simulink model "Overcurrent_Relay_design"  (R2024b)
settings: Solver=VariableStepAuto  StartTime=0.0  StopTime=0.4  RelTol=1e-3
undefined symbols (not defined in the file): D1, Delta
libraries: spsFourierLib x9, simulink x6, spsThreePhasePISectionLineLib x3, spsThreePhaseParallelRLCLoadLib x3, spsThreePhaseVIMeasurementLib x3, spsOnDelayLib x2, simulink_extras x2, spsThreePhaseBreakerLib x2, spsThreePhaseFaultLib x2, spsThreePhaseTransformerTwoWindingsLib x1, spsThreePhaseSourceLib x1, sps_lib x1
settings Model: Creator=Sabyasachi  LastModifiedBy=Sabyasachi

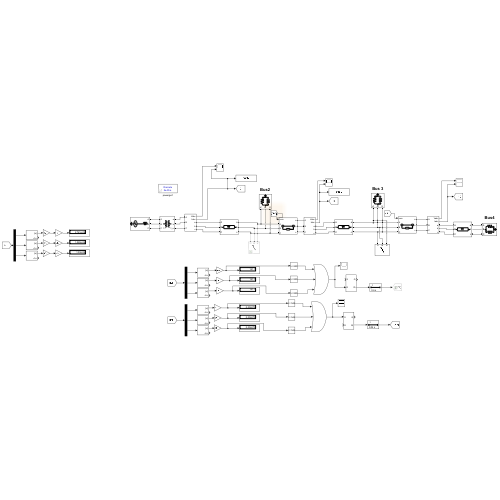
[thumbnail: Simulink's stored preview of the top-level diagram]
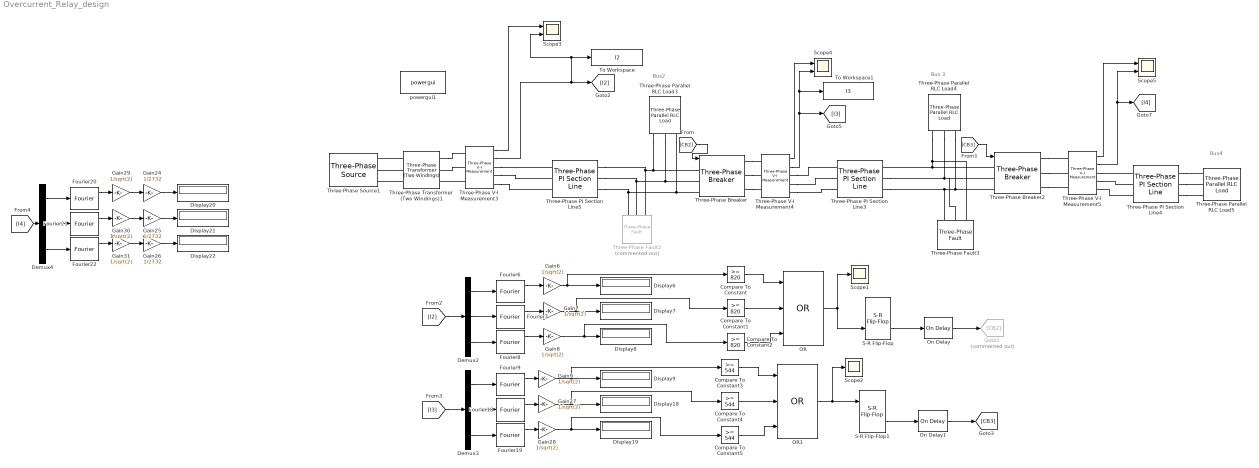
== system Overcurrent_Relay_design ==
  note: Bus4
  note: Bus 3
  note: Bus2
  Compare To Constant : simulink/Logic and Bit Operations/Compare To Constant  relop=>=  const=820  OutDataTypeStr=boolean
  Compare To Constant1 : simulink/Logic and Bit Operations/Compare To Constant  relop=>=  const=820  OutDataTypeStr=boolean
  Compare To Constant2 : simulink/Logic and Bit Operations/Compare To Constant  relop=>=  const=820  OutDataTypeStr=boolean
  Compare To Constant3 : simulink/Logic and Bit Operations/Compare To Constant  relop=>=  const=544  OutDataTypeStr=boolean
  Compare To Constant4 : simulink/Logic and Bit Operations/Compare To Constant  relop=>=  const=544  OutDataTypeStr=boolean
  Compare To Constant5 : simulink/Logic and Bit Operations/Compare To Constant  relop=>=  const=544  OutDataTypeStr=boolean
  Demux2 : Demux  Outputs=3
  Demux3 : Demux  Outputs=3
  Demux4 : Demux  Outputs=3
  Display{6..9,18..22} (9 alike) : Display
  Fourier{6..9,18..22} (9 alike) : spsFourierLib/Fourier  Freq=50  n=1  InInit=[0, 0]  Ts=0
  Gain24 : Gain  Gain=1/2732
  Gain25 : Gain  Gain=1/2732
  Gain26 : Gain  Gain=1/2732
  Gain{6..9,27..31} (9 alike) : Gain  Gain=1/sqrt(2)
  Goto1 : Goto  Commented=on  GotoTag=CB2
  OR : Logic  Operator=OR  Inputs=3  IconShape=distinctive  AllPortsSameDT=off  OutDataTypeStr=boolean
  OR1 : Logic  Operator=OR  Inputs=3  IconShape=distinctive  AllPortsSameDT=off  OutDataTypeStr=boolean
  On Delay : spsOnDelayLib/On Delay  DelayType=On delay  delay=0.6  ic=0  Ts=0
  On Delay1 : spsOnDelayLib/On Delay  DelayType=On delay  delay=0.04  ic=0  Ts=0
  S-R Flip-Flop : simulink_extras/Flip Flops/S-R Flip-Flop  initial_condition=0
  S-R Flip-Flop1 : simulink_extras/Flip Flops/S-R Flip-Flop  initial_condition=0
  Scope1 : Scope
  Scope2 : Scope
  Scope3 : Scope  NumInputPorts=2
  Scope4 : Scope  NumInputPorts=2
  Scope5 : Scope  NumInputPorts=2
  Three-Phase PI Section Line3 : spsThreePhasePISectionLineLib/Three-Phase PI Section Line  LConnTagsString=a|b|c  RConnTagsString=A|B|C  Length=1  Frequency=50  Resistances=[0.1486 0.2972]  Inductances=[4.73e-4 9.46e-4]  Capacitances=[1e-12 1e-12]
  Three-Phase PI Section Line4 : spsThreePhasePISectionLineLib/Three-Phase PI Section Line  LConnTagsString=a|b|c  RConnTagsString=A|B|C  Length=1  Frequency=50  Resistances=[0.1486 0.2972]  Inductances=[4.73e-4 9.46e-4]  Capacitances=[1e-12 1e-12]
  Three-Phase PI Section Line5 : spsThreePhasePISectionLineLib/Three-Phase PI Section Line  LConnTagsString=a|b|c  RConnTagsString=A|B|C  Length=1  Frequency=50  Resistances=[0.1486 0.2972]  Inductances=[4.73e-4 9.46e-4]  Capacitances=[1e-12 1e-12]
  Three-Phase Parallel RLC Load3 : spsThreePhaseParallelRLCLoadLib/Three-Phase Parallel RLC Load  LConnTagsString=A|B|C  Configuration=Y (grounded)  NominalVoltage=11e3  Vabc=[1e3 1e3 1e3]  Vabcp=[1e3 1e3 1e3]  NominalFrequency=50  UnbalancedPower=off  ActivePower=2.42e6  InductivePower=1.245e6  CapacitivePower=0  Pabc=[10e3 9e3 11e3]  QLabc=[100 90 110]  QCabc=[100 90 110]  Pabcp=[10e3 9e3 11e3]  QLabcp=[100 90 110]  QCabcp=[100 90 110]  Measurements=None  LoadType=constant Z
  Three-Phase Parallel RLC Load4 : spsThreePhaseParallelRLCLoadLib/Three-Phase Parallel RLC Load  LConnTagsString=A|B|C  Configuration=Y (grounded)  NominalVoltage=11e3  Vabc=[1e3 1e3 1e3]  Vabcp=[1e3 1e3 1e3]  NominalFrequency=50  UnbalancedPower=off  ActivePower=1.61e6  InductivePower=0.830e6  CapacitivePower=0  Pabc=[10e3 9e3 11e3]  QLabc=[100 90 110]  QCabc=[100 90 110]  Pabcp=[10e3 9e3 11e3]  QLabcp=[100 90 110]  QCabcp=[100 90 110]  Measurements=None  LoadType=constant Z
  Three-Phase Parallel RLC Load5 : spsThreePhaseParallelRLCLoadLib/Three-Phase Parallel RLC Load  LConnTagsString=A|B|C  Configuration=Y (grounded)  NominalVoltage=11e3  Vabc=[1e3 1e3 1e3]  Vabcp=[1e3 1e3 1e3]  NominalFrequency=50  UnbalancedPower=off  ActivePower=3.23e6  InductivePower=1.660e6  CapacitivePower=0  Pabc=[10e3 9e3 11e3]  QLabc=[100 90 110]  QCabc=[100 90 110]  Pabcp=[10e3 9e3 11e3]  QLabcp=[100 90 110]  QCabcp=[100 90 110]  Measurements=None  LoadType=constant Z
  Three-Phase Transformer (Two Windings)1 : spsThreePhaseTransformerTwoWindingsLib/Three-Phase Transformer (Two Windings)  Winding1Connection=Delta (D1)  Winding2Connection=Yg  CoreType=Three single-phase transformers  SetSaturation=off  Hysteresis=off  DataFile='hysteresis'  SetInitialFlux=off  Measurements=None  UNITS=pu  NominalPower=[ 17e6 , 50 ]  Winding1=[33e3 , 1e-6 , 0.05 ]  Winding2=[ 11e3 , 1e-6 , 1e-6 ]  Rm=500  Lm=500  L0=0.5  Saturation=[ 0,0 ; 0.0024,1.2 ; 1.0,1.52 ]  InitialFluxes=[ 0.8 , -0.8 , 0.7 ]  BreakLoop=off  DiscreteSolver=Trapezoidal iterative  DataType=off  TransfoNumber=1
  Three-Phase V-I Measurement3 : spsThreePhaseVIMeasurementLib/Three-Phase V-I Measurement  VoltageMeasurement=phase-to-ground  SetLabelV=off  LabelV=Vabc  Vpu=off  VpuLL=off  CurrentMeasurement=yes  SetLabelI=off  LabelI=Iabc  Ipu=off  Pbase=100e6  Vbase=500e3  OutputType=Complex  PhasorSimulation=off  PSBequivalent=0
  Three-Phase V-I Measurement4 : spsThreePhaseVIMeasurementLib/Three-Phase V-I Measurement  VoltageMeasurement=phase-to-ground  SetLabelV=off  LabelV=Vabc  Vpu=off  VpuLL=off  CurrentMeasurement=yes  SetLabelI=off  LabelI=Iabc  Ipu=off  Pbase=100e6  Vbase=500e3  OutputType=Complex  PhasorSimulation=off  PSBequivalent=0
  Three-Phase V-I Measurement5 : spsThreePhaseVIMeasurementLib/Three-Phase V-I Measurement  VoltageMeasurement=phase-to-ground  SetLabelV=off  LabelV=Vabc  Vpu=off  VpuLL=off  CurrentMeasurement=yes  SetLabelI=off  LabelI=Iabc  Ipu=off  Pbase=100e6  Vbase=500e3  OutputType=Complex  PhasorSimulation=off  PSBequivalent=0
  Three-Phase Breaker : spsThreePhaseBreakerLib/Three-Phase Breaker  InitialState=closed  SwitchA=on  SwitchB=on  SwitchC=on  SwitchTimes="[1/60  5/60]"  External=on  BreakerResistance=0.01  SnubberResistance=1e6  SnubberCapacitance=inf  Measurements=None
  Three-Phase Breaker2 : spsThreePhaseBreakerLib/Three-Phase Breaker  InitialState=closed  SwitchA=on  SwitchB=on  SwitchC=on  SwitchTimes="[1/60  5/60]"  External=on  BreakerResistance=0.01  SnubberResistance=1e6  SnubberCapacitance=inf  Measurements=None
  Three-Phase Fault2 : spsThreePhaseFaultLib/Three-Phase Fault  Commented=on  InitialStates=0  FaultA=on  FaultB=off  FaultC=off  GroundFault=on  SwitchTimes=[0.2]  External=off  SwitchStatus=NaN  FaultResistance=0.001  GroundResistance=0.01  SnubberResistance=1e6  SnubberCapacitance=inf  Measurements=None
  Three-Phase Fault3 : spsThreePhaseFaultLib/Three-Phase Fault  InitialStates=0  FaultA=on  FaultB=off  FaultC=off  GroundFault=on  SwitchTimes=[0.2]  External=off  SwitchStatus=NaN  FaultResistance=0.001  GroundResistance=0.01  SnubberResistance=1e6  SnubberCapacitance=inf  Measurements=None
  Three-Phase Source1 : spsThreePhaseSourceLib/Three-Phase Source  InternalConnection=Yg  VoltagePhases=off  Voltage=33e3  PhaseAngle=0  Voltage_phases=[25e3 25e3 25e3]/sqrt(3)  PhaseAngles_phases=[0 -120 +120]  Frequency=50  NonIdealSource=on  SpecifyImpedance=off  Resistance=0  Inductance=0.01  ShortCircuitLevel=100e6  BaseVoltage=33e3  XRratio=7  BusType=swing  Pref=10e3  Qref=0  Prefabc=[10e3, 10e3, 10e3]  Qrefabc=[0, 0, 0]  Qmin=-inf  Qmax=inf
  To Workspace : ToWorkspace  VariableName=I2  SaveFormat=Timeseries  SampleTime=-1
  To Workspace1 : ToWorkspace  VariableName=I3  SaveFormat=Timeseries  SampleTime=-1
  powergui1 : sps_lib/powergui  Priority=1  SimulationMode=Discrete  SampleTime=50e-6  frequency=50  Iterations=50  frequencyindice=50  Pbase=100e6  ErrMax=1e-4  UnitsV=kV  UnitsW=MW  buscounter=0  FunctionMessages=off  echomessages=off  EnableUseOfTLC=off  CurrentSourceSwitches=off  DisableSnubberDevices=off  DisableRonSwitches=off  DisableVfSwitches=off  DisplayEquations=off  AutomaticDiscreteSolvers=off  SolverType=Tustin/Backward Euler (TBE)  Interpol=off  ExternalGateDelay=off  methode=off  Ts=100  x0status=blocks  SPID=on  SwTol=0  HookPort=off  NonlinearTolerance=1e-4  nMaxIteration=100  ContinueOnMaxIteration=off  RestoreLinks=warning  ResistiveCurrentMeasurement=off  Frange=[0:2:500]  Ylog=off  Xlog=on  ShowGrid=off  save=off  variable=ZData  structure=0  ZoomFFT=off  StartTime=0.0  cycles=1  DisplayStyle=1  fundamental=60  FreqAxis=off  MaxFrequency=1000  frequencyindicesteady=1  RmsSteady=1  display=off
  wires:
  Gain29/1 -> Gain24/1
  [I4] -> Demux4/1
  Demux2/3 -> Fourier8/1
  Three-Phase V-I Measurement3/1 -> Scope3/1
  Gain31/1 -> Gain26/1
  Fourier7/1 -> Gain7/1
  Demux4/2 -> Fourier21/1
  Demux4/1 -> Fourier20/1
  Fourier20/1 -> Gain29/1
  [I2] -> Demux2/1
  Demux2/2 -> Fourier7/1
  Fourier21/1 -> Gain30/1
  Three-Phase V-I Measurement3/2 -> To Workspace/1, Scope3/2, [I2]
  Three-Phase V-I Measurement4/1 -> Scope4/1
  Gain25/1 -> Display21/1
  Three-Phase V-I Measurement5/2 -> Scope5/2, [I4]
  Fourier6/1 -> Gain6/1
  Fourier22/1 -> Gain31/1
  Three-Phase V-I Measurement4/2 -> Scope4/2, To Workspace1/1, [I3]
  Demux2/1 -> Fourier6/1
  Fourier8/1 -> Gain8/1
  Gain24/1 -> Display20/1
  Demux4/3 -> Fourier22/1
  Three-Phase V-I Measurement5/1 -> Scope5/1
  Gain26/1 -> Display22/1
  Gain30/1 -> Gain25/1
  OR/1 -> Scope1/1, S-R Flip-Flop/2
  Compare To Constant2/1 -> OR/3
  Compare To Constant1/1 -> OR/2
  Gain6/1 -> Compare To Constant/1, Display6/1
  On Delay/1 -> Goto1/1
  S-R Flip-Flop/2 -> On Delay/1
  Gain7/1 -> Compare To Constant1/1, Display7/1
  Gain8/1 -> Compare To Constant2/1, Display8/1
  Compare To Constant/1 -> OR/1
  Demux3/1 -> Fourier9/1
  Fourier9/1 -> Gain9/1
  Demux3/2 -> Fourier18/1
  Fourier18/1 -> Gain27/1
  Demux3/3 -> Fourier19/1
  Fourier19/1 -> Gain28/1
  [I3] -> Demux3/1
  Compare To Constant3/1 -> OR1/1
  Gain28/1 -> Compare To Constant5/1, Display19/1
  Gain27/1 -> Compare To Constant4/1, Display18/1
  S-R Flip-Flop1/2 -> On Delay1/1
  On Delay1/1 -> [CB3]
  Gain9/1 -> Compare To Constant3/1, Display9/1
  Compare To Constant4/1 -> OR1/2
  Compare To Constant5/1 -> OR1/3
  OR1/1 -> Scope2/1, S-R Flip-Flop1/1
  [CB2] -> Three-Phase Breaker/1
  [CB3] -> Three-Phase Breaker2/1
  connections:
  Three-Phase Parallel RLC Load4/LConn1 -- Three-Phase Fault3/LConn1 -- Three-Phase PI Section Line3/RConn1 -- Three-Phase Breaker2/LConn1
  Three-Phase Parallel RLC Load4/LConn2 -- Three-Phase PI Section Line3/RConn2 -- Three-Phase Breaker2/LConn2 -- Three-Phase Fault3/LConn2
  Three-Phase Parallel RLC Load4/LConn3 -- Three-Phase Fault3/LConn3 -- Three-Phase PI Section Line3/RConn3 -- Three-Phase Breaker2/LConn3
  Three-Phase PI Section Line4/LConn3 -- Three-Phase V-I Measurement5/RConn3
  Three-Phase PI Section Line4/RConn3 -- Three-Phase Parallel RLC Load5/LConn3
  Three-Phase PI Section Line4/RConn2 -- Three-Phase Parallel RLC Load5/LConn2
  Three-Phase Transformer (Two Windings)1/LConn2 -- Three-Phase Source1/RConn2
  Three-Phase PI Section Line4/LConn1 -- Three-Phase V-I Measurement5/RConn1
  Three-Phase V-I Measurement3/LConn2 -- Three-Phase Transformer (Two Windings)1/RConn2
  Three-Phase PI Section Line4/RConn1 -- Three-Phase Parallel RLC Load5/LConn1
  Three-Phase PI Section Line4/LConn2 -- Three-Phase V-I Measurement5/RConn2
  Three-Phase V-I Measurement3/LConn3 -- Three-Phase Transformer (Two Windings)1/RConn3
  Three-Phase Transformer (Two Windings)1/LConn1 -- Three-Phase Source1/RConn1
  Three-Phase Transformer (Two Windings)1/LConn3 -- Three-Phase Source1/RConn3
  Three-Phase Transformer (Two Windings)1/RConn1 -- Three-Phase V-I Measurement3/LConn1
  Three-Phase V-I Measurement3/RConn1 -- Three-Phase PI Section Line5/LConn1
  Three-Phase V-I Measurement3/RConn2 -- Three-Phase PI Section Line5/LConn2
  Three-Phase V-I Measurement3/RConn3 -- Three-Phase PI Section Line5/LConn3
  Three-Phase Breaker/RConn1 -- Three-Phase V-I Measurement4/LConn1
  Three-Phase Breaker/RConn2 -- Three-Phase V-I Measurement4/LConn2
  Three-Phase Breaker/RConn3 -- Three-Phase V-I Measurement4/LConn3
  Three-Phase PI Section Line5/RConn1 -- Three-Phase Fault2/LConn1 -- Three-Phase Parallel RLC Load3/LConn1 -- Three-Phase Breaker/LConn1
  Three-Phase PI Section Line5/RConn2 -- Three-Phase Fault2/LConn2 -- Three-Phase Parallel RLC Load3/LConn2 -- Three-Phase Breaker/LConn2
  Three-Phase PI Section Line5/RConn3 -- Three-Phase Fault2/LConn3 -- Three-Phase Parallel RLC Load3/LConn3 -- Three-Phase Breaker/LConn3
  Three-Phase V-I Measurement4/RConn1 -- Three-Phase PI Section Line3/LConn1
  Three-Phase V-I Measurement4/RConn2 -- Three-Phase PI Section Line3/LConn2
  Three-Phase V-I Measurement4/RConn3 -- Three-Phase PI Section Line3/LConn3
  Three-Phase Breaker2/RConn1 -- Three-Phase V-I Measurement5/LConn1
  Three-Phase Breaker2/RConn2 -- Three-Phase V-I Measurement5/LConn2
  Three-Phase Breaker2/RConn3 -- Three-Phase V-I Measurement5/LConn3
